simulink model "lookup_table"  (R2018b)
settings: Solver=FixedStepAuto  StartTime=0.0  StopTime=8  FixedStep=1  RelTol=1e-3
undefined symbols (not defined in the file or in its folder): VarName1, VarName2
libraries: simulink x2
settings Model: Creator=marwan  LastModifiedBy=marwan

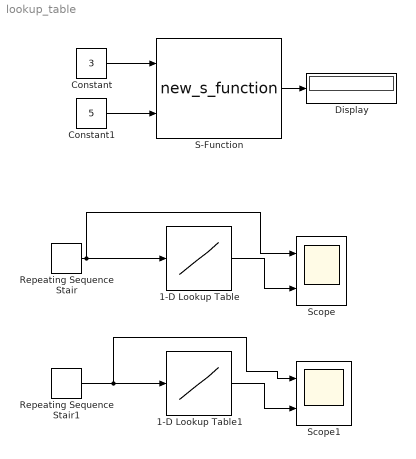
== system lookup_table ==
  1-D Lookup Table : Lookup_n-D  NumberOfTableDimensions=1  BreakpointsForDimension1=[0.5:0.04:4.5]  Table=[0:1:100]  InternalRulePriority=Speed  RndMeth=Simplest  InputSameDT=on
  1-D Lookup Table1 : Lookup_n-D  NumberOfTableDimensions=1  BreakpointsForDimension1=VarName2  Table=VarName1  InternalRulePriority=Speed  RndMeth=Simplest  InputSameDT=on
  Constant : Constant  Value=3
  Constant1 : Constant  Value=5
  Display : Display
      settings: Decimation=2
  Repeating Sequence Stair : simulink/Sources/Repeating Sequence Stair  OutValues=sens  tsamp=-1  OutMin=[]  OutMax=[]  OutDataTypeStr=double  OutputDataTypeScalingMode=double  OutDataType=fixdt(0,8)  ConRadixGroup=Best Precision: Vector-wise  OutScaling=2^-12
  Repeating Sequence Stair1 : simulink/Sources/Repeating Sequence Stair  OutValues=sens  tsamp=-1  OutMin=[]  OutMax=[]  OutDataTypeStr=double  OutputDataTypeScalingMode=double  OutDataType=fixdt(0,8)  ConRadixGroup=Best Precision: Vector-wise  OutScaling=2^-12
  S-Function : S-Function  FunctionName=new_s_function  SFunctionDeploymentMode=off  EnableBusSupport=off
  Scope : Scope  NumInputPorts=2
  Scope1 : Scope  NumInputPorts=2
  wires:
  Constant/1 -> S-Function/1
  Constant1/1 -> S-Function/2
  S-Function/1 -> Display/1
  Repeating Sequence Stair1/1 -> Scope1/1, 1-D Lookup Table1/1
  1-D Lookup Table/1 -> Scope/2
  Repeating Sequence Stair/1 -> Scope/1, 1-D Lookup Table/1
  1-D Lookup Table1/1 -> Scope1/2
